simulink model "ACC_HW"  (R2017a)
settings: Solver=ode2  StartTime=0.0  StopTime=endTime  FixedStep=Ts  RelTol=1e-3
undefined symbols (not defined in the file): Ts, v0_host, v0_lead, vref_host, x0_host, x0_lead
settings Model: Creator=jyotirmoy  LastModifiedBy=jyotirmoy

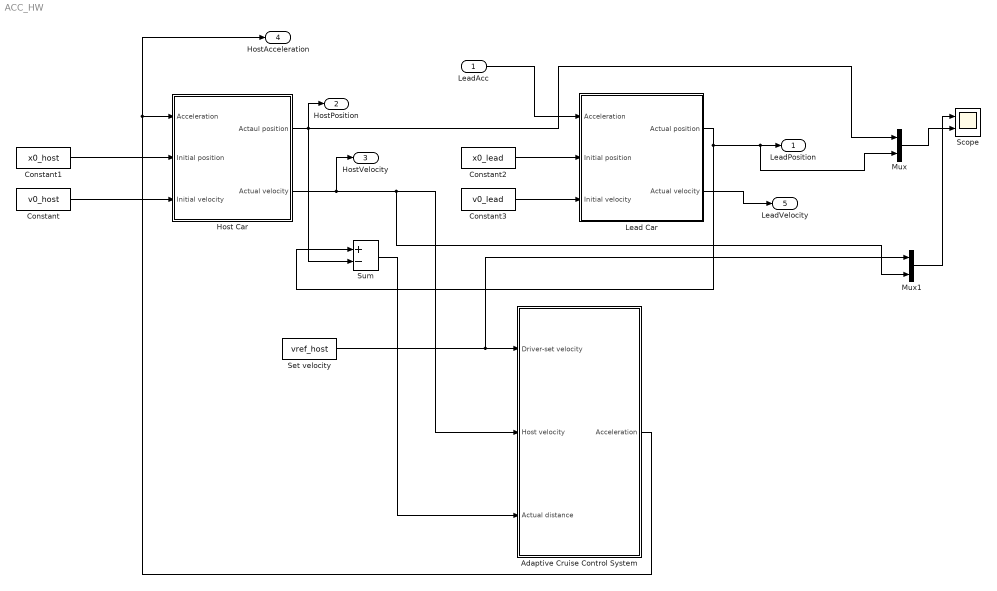
== system ACC_HW ==
  LeadAcc : Inport
  Adaptive Cruise Control System : Subsystem  VariantControl=MODE==4
  Constant : Constant  Value=v0_host
  Constant1 : Constant  Value=x0_host
  Constant2 : Constant  Value=x0_lead
  Constant3 : Constant  Value=v0_lead
  Host Car : Subsystem
  Lead Car : Subsystem
  Mux : Mux  Inputs=2
  Mux1 : Mux  Inputs=2
  Scope : Scope  NumInputPorts=2
  Set velocity : Constant  Value=vref_host  SampleTime=Ts
  Sum : Sum  Inputs=+-
  LeadPosition : Outport
  HostPosition : Outport  Port=2
  HostVelocity : Outport  Port=3
  HostAcceleration : Outport  Port=4
  LeadVelocity : Outport  Port=5
  wires:
  Host Car/1(Actaul position) -> Mux/1, Sum/2, HostPosition/1
  Set velocity/1 -> Mux1/1, Adaptive Cruise Control System/1(Driver-set velocity)
  Sum/1 -> Adaptive Cruise Control System/3(Actual distance)
  Host Car/2(Actual velocity) -> HostVelocity/1, Mux1/2, Adaptive Cruise Control System/2(Host velocity)
  Constant/1 -> Host Car/3(Initial velocity)
  Constant1/1 -> Host Car/2(Initial position)
  Adaptive Cruise Control System/1("Acceleration ") -> HostAcceleration/1, Host Car/1(Acceleration)
  Constant2/1 -> Lead Car/2(Initial position)
  Constant3/1 -> Lead Car/3(Initial velocity)
  LeadAcc/1 -> Lead Car/1(Acceleration)
  Lead Car/1(Actual position) -> Mux/2, LeadPosition/1, Sum/1
  Mux/1 -> Scope/2
  Mux1/1 -> Scope/1
  Lead Car/2(Actual velocity) -> LeadVelocity/1

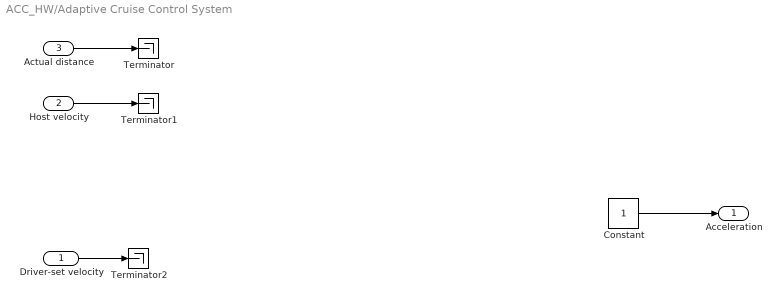
== system ACC_HW/Adaptive Cruise Control System ==
  Driver-set velocity : Inport
  Host velocity : Inport  Port=2
  Actual distance : Inport  Port=3
  Constant : Constant
  Terminator : Terminator
  Terminator1 : Terminator
  Terminator2 : Terminator
  "Acceleration " : Outport
  wires:
  Driver-set velocity/1 -> Terminator2/1
  Actual distance/1 -> Terminator/1
  Host velocity/1 -> Terminator1/1
  Constant/1 -> "Acceleration "/1

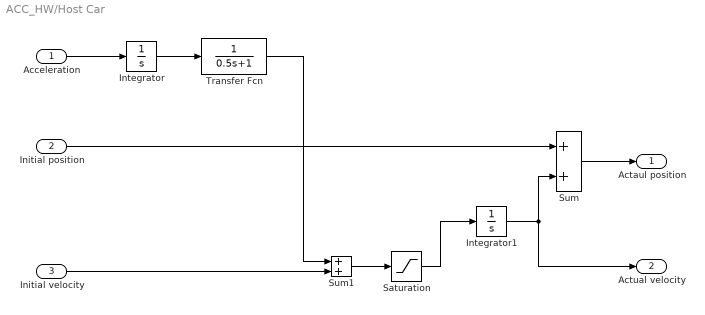
== system ACC_HW/Host Car ==
  Acceleration : Inport
  Initial position : Inport  Port=2
  Initial velocity : Inport  Port=3
  Integrator : Integrator
  Integrator1 : Integrator
  Saturation : Saturate  UpperLimit=60  LowerLimit=0
  Sum : Sum
  Sum1 : Sum
  Transfer Fcn : TransferFcn  Denominator=[0.5 1]
  Actaul position : Outport
  Actual velocity : Outport  Port=2
  wires:
  Initial velocity/1 -> Sum1/2
  Sum/1 -> Actaul position/1
  Transfer Fcn/1 -> Sum1/1
  Integrator/1 -> Transfer Fcn/1
  Acceleration/1 -> Integrator/1
  Initial position/1 -> Sum/1
  Integrator1/1 -> Sum/2, Actual velocity/1
  Sum1/1 -> Saturation/1
  Saturation/1 -> Integrator1/1

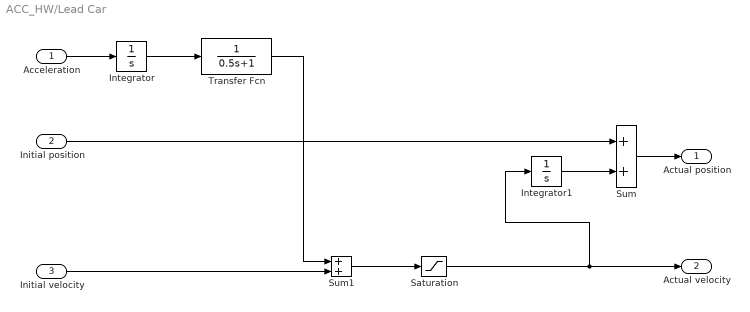
== system ACC_HW/Lead Car ==
  Acceleration : Inport
  Initial position : Inport  Port=2
  Initial velocity : Inport  Port=3
  Integrator : Integrator
  Integrator1 : Integrator
  Saturation : Saturate  UpperLimit=60  LowerLimit=0
  Sum : Sum
  Sum1 : Sum
  Transfer Fcn : TransferFcn  Denominator=[0.5 1]
  Actual position : Outport
  Actual velocity : Outport  Port=2
  wires:
  Transfer Fcn/1 -> Sum1/1
  Initial velocity/1 -> Sum1/2
  Sum/1 -> Actual position/1
  Integrator/1 -> Transfer Fcn/1
  Acceleration/1 -> Integrator/1
  Initial position/1 -> Sum/1
  Integrator1/1 -> Sum/2
  Saturation/1 -> Integrator1/1, Actual velocity/1
  Sum1/1 -> Saturation/1
